simulink model "Requirements_Table"  (R2022a)
settings: Solver=FixedStepAuto  StartTime=0.0  StopTime=10.0  FixedStep=1e-3  RelTol=1e-3  EnableMultiTasking=on
settings Model: ExtModeTrigDuration=5  Creator=sabri  LastModifiedBy=Tim
settings SolverCC: AlgebraicLoopSolver=TrustRegion
settings OptimizationCC: EnhancedBackFolding=on  PassReuseOutputArgsAs=Individual arguments  ZeroExternalMemoryAtStartup=off  ZeroInternalMemoryAtStartup=off  MaxStackSize=64  OptimizeBlockOrder=speed  DifferentSizesBufferReuse=on  OptimizationCustomize=off  EfficientTunableParamExpr=on
settings DebuggingCC: ParameterTunabilityLossMsg=error  UnconnectedInputMsg=warning  UnconnectedOutputMsg=warning  UnconnectedLineMsg=warning  SFMachineParentedDataDiag=warning
settings HardwareCC: ProdBitPerPointer=32  ProdBitPerSizeT=32  ProdBitPerPtrDiffT=32  ProdLargestAtomicInteger=Long  ProdLargestAtomicFloat=Double  ProdWordSize=32  ProdHWDeviceType=ARM Compatible->ARM Cortex
settings SFSimCC: MATLABDynamicMemAlloc=off
settings RTWCC: SystemTargetFile=ert.tlc  HardwareBoard=NXP FRDM-K64F  TLCOptions="-aInlineSetEventsForThisBaseRateFcn=TLC_FALSE -aSuppressMultiTaskScheduler=TLC_FALSE  -aRateBasedStepFcn=0"  TemplateMakefile=ert_default_tmf  Toolchain=GNU Tools for ARM Embedded Processors
settings CodeAppCC: ForceParamTrailComments=on  IgnoreCustomStorageClasses=off  OperatorAnnotations=on  SimulinkDataObjDesc=on  SFDataObjDesc=on  InsertBlockDesc=on

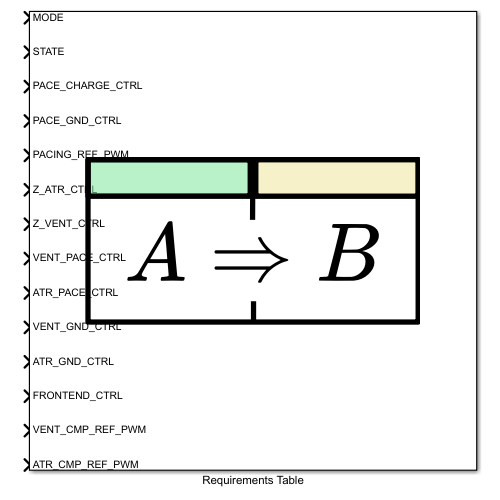
[thumbnail: Simulink's stored preview of the top-level diagram]
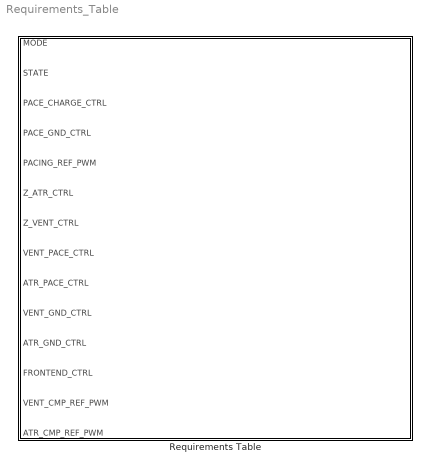
== system Requirements_Table ==
  Requirements Table : Requirements Table  TreatAsAtomicUnit=on

== stateflow chart Requirements_Table/Requirements Table ==
  (default) -> (junction 1073754062)
  (junction 1073754062) -> (junction 1073754063) : {
      | % SF_REQ_REV_07
      | }
  (junction 1073754063) -> (junction 1073754065) : {
      | % HEADER_ASSIGNMENTS
      |
      | }
  (junction 1073754065) -> (junction 1073754067) : {
      | % START_A_4
      | }
  (junction 1073754067) -> (junction 1073754069) : {
      | }
  (junction 1073754069) -> (junction 1073754071)
  (junction 1073754071) -> (junction 1073754073) : {
      | }
  (junction 1073754073) -> (junction 1073754075) : {
      | % END_A_4
      | }
  (junction 1073754075) -> (junction 1073754077) : {
      | % START_R_1
      | }
  (junction 1073754077) -> (junction 1073754079) : {
      | }
  (junction 1073754079) -> (junction 1073754081)
  (junction 1073754081) -> (junction 1073754083) [order 1] : [(((MODE) == (1)))]
  (junction 1073754081) -> (junction 1073754125) [order 2]
  (junction 1073754083) -> (junction 1073754085) : {
      | reqtable_postcondition((((FRONTEND_CTRL) == (0))), 'R:1');
      |
      |
      | }
  (junction 1073754085) -> (junction 1073754087) : {
      | }
  (junction 1073754087) -> (junction 1073754089) : {
      | % START_R_10
      | }
  (junction 1073754089) -> (junction 1073754091) : {
      | }
  (junction 1073754091) -> (junction 1073754093)
  (junction 1073754093) -> (junction 1073754095) [order 1] : [(((STATE) == (1)))]
  (junction 1073754093) -> (junction 1073754101) [order 2]
  (junction 1073754095) -> (junction 1073754097) : {
      | reqtable_postcondition((((PACE_CHARGE_CTRL) == (0))) && (((PACE_GND_CTRL) == (1))) && (((PACING_REF_PWM) == (vent_amp))) && (((Z_ATR_CTRL) == (0))) && (((Z_VENT_CTRL) == (0))) && (((VENT_PACE_CTRL) == (1))) && (((ATR_PACE_CTRL) == (0))) && (((VENT_GND_CTRL) == (0))) && (((ATR_GND_CTRL) == (0))), 'R:1.1');
      |
      |
      | }
  (junction 1073754097) -> (junction 1073754099) : {
      | }
  (junction 1073754099) -> (junction 1073754101)
  (junction 1073754101) -> (junction 1073754103)
  (junction 1073754103) -> (junction 1073754105) : {
      | % END_R_10
      | }
  (junction 1073754105) -> (junction 1073754107) : {
      | % START_R_16
      | }
  (junction 1073754107) -> (junction 1073754109) : {
      | }
  (junction 1073754109) -> (junction 1073754111)
  (junction 1073754111) -> (junction 1073754113) [order 1] : [(((STATE) == (0)))]
  (junction 1073754111) -> (junction 1073754119) [order 2]
  (junction 1073754113) -> (junction 1073754115) : {
      | reqtable_postcondition((((PACE_CHARGE_CTRL) == (1))) && (((PACE_GND_CTRL) == (1))) && (((PACING_REF_PWM) == (vent_amp))) && (((Z_ATR_CTRL) == (0))) && (((Z_VENT_CTRL) == (0))) && (((VENT_PACE_CTRL) == (0))) && (((ATR_PACE_CTRL) == (0))) && (((VENT_GND_CTRL) == (1))) && (((ATR_GND_CTRL) == (0))), 'R:1.2');
      |
      |
      | }
  (junction 1073754115) -> (junction 1073754117) : {
      | }
  (junction 1073754117) -> (junction 1073754119)
  (junction 1073754119) -> (junction 1073754121)
  (junction 1073754121) -> (junction 1073754123) : {
      | % END_R_16
      | }
  (junction 1073754123) -> (junction 1073754125)
  (junction 1073754125) -> (junction 1073754127)
  (junction 1073754127) -> (junction 1073754129) : {
      | % END_R_1
      | }
  (junction 1073754129) -> (junction 1073754131) : {
      | % START_R_7
      | }
  (junction 1073754131) -> (junction 1073754133) : {
      | }
  (junction 1073754133) -> (junction 1073754135)
  (junction 1073754135) -> (junction 1073754137) [order 1] : [(((MODE) == (2)))]
  (junction 1073754135) -> (junction 1073754179) [order 2]
  (junction 1073754137) -> (junction 1073754139) : {
      | reqtable_postcondition((((FRONTEND_CTRL) == (0))), 'R:2');
      |
      |
      | }
  (junction 1073754139) -> (junction 1073754141) : {
      | }
  (junction 1073754141) -> (junction 1073754143) : {
      | % START_R_19
      | }
  (junction 1073754143) -> (junction 1073754145) : {
      | }
  (junction 1073754145) -> (junction 1073754147)
  (junction 1073754147) -> (junction 1073754149) [order 1] : [(((STATE) == (1)))]
  (junction 1073754147) -> (junction 1073754155) [order 2]
  (junction 1073754149) -> (junction 1073754151) : {
      | reqtable_postcondition((((PACE_CHARGE_CTRL) == (0))) && (((PACE_GND_CTRL) == (1))) && (((PACING_REF_PWM) == (atr_amp))) && (((Z_ATR_CTRL) == (0))) && (((Z_VENT_CTRL) == (0))) && (((VENT_PACE_CTRL) == (0))) && (((ATR_PACE_CTRL) == (1))) && (((VENT_GND_CTRL) == (0))) && (((ATR_GND_CTRL) == (0))), 'R:2.1');
      |
      |
      | }
  (junction 1073754151) -> (junction 1073754153) : {
      | }
  (junction 1073754153) -> (junction 1073754155)
  (junction 1073754155) -> (junction 1073754157)
  (junction 1073754157) -> (junction 1073754159) : {
      | % END_R_19
      | }
  (junction 1073754159) -> (junction 1073754161) : {
      | % START_R_25
      | }
  (junction 1073754161) -> (junction 1073754163) : {
      | }
  (junction 1073754163) -> (junction 1073754165)
  (junction 1073754165) -> (junction 1073754167) [order 1] : [(((STATE) == (0)))]
  (junction 1073754165) -> (junction 1073754173) [order 2]
  (junction 1073754167) -> (junction 1073754169) : {
      | reqtable_postcondition((((PACE_CHARGE_CTRL) == (1))) && (((PACE_GND_CTRL) == (1))) && (((PACING_REF_PWM) == (atr_amp))) && (((Z_ATR_CTRL) == (0))) && (((Z_VENT_CTRL) == (0))) && (((VENT_PACE_CTRL) == (0))) && (((ATR_PACE_CTRL) == (0))) && (((VENT_GND_CTRL) == (0))) && (((ATR_GND_CTRL) == (1))), 'R:2.2');
      |
      |
      | }
  (junction 1073754169) -> (junction 1073754171) : {
      | }
  (junction 1073754171) -> (junction 1073754173)
  (junction 1073754173) -> (junction 1073754175)
  (junction 1073754175) -> (junction 1073754177) : {
      | % END_R_25
      | }
  (junction 1073754177) -> (junction 1073754179)
  (junction 1073754179) -> (junction 1073754181)
  (junction 1073754181) -> (junction 1073754183) : {
      | % END_R_7
      | }
  (junction 1073754183) -> (junction 1073754185) : {
      | % START_R_28
      | }
  (junction 1073754185) -> (junction 1073754187) : {
      | }
  (junction 1073754187) -> (junction 1073754189)
  (junction 1073754189) -> (junction 1073754191) [order 1] : [(((MODE) == (3)))]
  (junction 1073754189) -> (junction 1073754251) [order 2]
  (junction 1073754191) -> (junction 1073754193) : {
      |
      |
      | }
  (junction 1073754193) -> (junction 1073754195) : {
      | }
  (junction 1073754195) -> (junction 1073754197) : {
      | % START_R_34
      | }
  (junction 1073754197) -> (junction 1073754199) : {
      | }
  (junction 1073754199) -> (junction 1073754201)
  (junction 1073754201) -> (junction 1073754203) [order 1] : [(((STATE) == (1)))]
  (junction 1073754201) -> (junction 1073754209) [order 2]
  (junction 1073754203) -> (junction 1073754205) : {
      | reqtable_postcondition((((PACE_CHARGE_CTRL) == (0))) && (((PACE_GND_CTRL) == (1))) && (((PACING_REF_PWM) == (vent_amp))) && (((Z_ATR_CTRL) == (0))) && (((Z_VENT_CTRL) == (0))) && (((VENT_PACE_CTRL) == (1))) && (((ATR_PACE_CTRL) == (0))) && (((VENT_GND_CTRL) == (0))) && (((ATR_GND_CTRL) == (0))), 'R:3.1');
      |
      |
      | }
  (junction 1073754205) -> (junction 1073754207) : {
      | }
  (junction 1073754207) -> (junction 1073754209)
  (junction 1073754209) -> (junction 1073754211)
  (junction 1073754211) -> (junction 1073754213) : {
      | % END_R_34
      | }
  (junction 1073754213) -> (junction 1073754215) : {
      | % START_R_37
      | }
  (junction 1073754215) -> (junction 1073754217) : {
      | }
  (junction 1073754217) -> (junction 1073754219)
  (junction 1073754219) -> (junction 1073754221) [order 1] : [(((STATE) == (0)))]
  (junction 1073754219) -> (junction 1073754227) [order 2]
  (junction 1073754221) -> (junction 1073754223) : {
      | reqtable_postcondition((((PACE_CHARGE_CTRL) == (1))) && (((PACE_GND_CTRL) == (1))) && (((PACING_REF_PWM) == (vent_amp))) && (((Z_ATR_CTRL) == (0))) && (((Z_VENT_CTRL) == (0))) && (((VENT_PACE_CTRL) == (0))) && (((ATR_PACE_CTRL) == (0))) && (((VENT_GND_CTRL) == (1))) && (((ATR_GND_CTRL) == (0))) && (((FRONTEND_CTRL) == (1))), 'R:3.2');
      |
      |
      | }
  (junction 1073754223) -> (junction 1073754225) : {
      | }
  (junction 1073754225) -> (junction 1073754227)
  (junction 1073754227) -> (junction 1073754229)
  (junction 1073754229) -> (junction 1073754231) : {
      | % END_R_37
      | }
  (junction 1073754231) -> (junction 1073754233) : {
      | % START_R_40
      | }
  (junction 1073754233) -> (junction 1073754235) : {
      | }
  (junction 1073754235) -> (junction 1073754237)
  (junction 1073754237) -> (junction 1073754239) [order 1] : [(((STATE) == (2)))]
  (junction 1073754237) -> (junction 1073754245) [order 2]
  (junction 1073754239) -> (junction 1073754241) : {
      | reqtable_postcondition((((PACE_CHARGE_CTRL) == (1))) && (((PACE_GND_CTRL) == (1))) && (((PACING_REF_PWM) == (vent_amp))) && (((Z_ATR_CTRL) == (0))) && (((Z_VENT_CTRL) == (0))) && (((VENT_PACE_CTRL) == (0))) && (((ATR_PACE_CTRL) == (0))) && (((VENT_GND_CTRL) == (1))) && (((ATR_GND_CTRL) == (0))) && (((FRONTEND_CTRL) == (0))), 'R:3.3');
      |
      |
      | }
  (junction 1073754241) -> (junction 1073754243) : {
      | }
  (junction 1073754243) -> (junction 1073754245)
  (junction 1073754245) -> (junction 1073754247)
  (junction 1073754247) -> (junction 1073754249) : {
      | % END_R_40
      | }
  (junction 1073754249) -> (junction 1073754251)
  (junction 1073754251) -> (junction 1073754253)
  (junction 1073754253) -> (junction 1073754255) : {
      | % END_R_28
      | }
  (junction 1073754255) -> (junction 1073754257) : {
      | % START_R_31
      | }
  (junction 1073754257) -> (junction 1073754259) : {
      | }
  (junction 1073754259) -> (junction 1073754261)
  (junction 1073754261) -> (junction 1073754263) [order 1] : [(((MODE) == (4)))]
  (junction 1073754261) -> (junction 1073754323) [order 2]
  (junction 1073754263) -> (junction 1073754265) : {
      |
      |
      | }
  (junction 1073754265) -> (junction 1073754267) : {
      | }
  (junction 1073754267) -> (junction 1073754269) : {
      | % START_R_52
      | }
  (junction 1073754269) -> (junction 1073754271) : {
      | }
  (junction 1073754271) -> (junction 1073754273)
  (junction 1073754273) -> (junction 1073754275) [order 1] : [(((STATE) == (1)))]
  (junction 1073754273) -> (junction 1073754281) [order 2]
  (junction 1073754275) -> (junction 1073754277) : {
      | reqtable_postcondition((((PACE_CHARGE_CTRL) == (0))) && (((PACE_GND_CTRL) == (1))) && (((PACING_REF_PWM) == (atr_amp))) && (((Z_ATR_CTRL) == (0))) && (((Z_VENT_CTRL) == (0))) && (((VENT_PACE_CTRL) == (0))) && (((ATR_PACE_CTRL) == (1))) && (((VENT_GND_CTRL) == (0))) && (((ATR_GND_CTRL) == (0))), 'R:4.1');
      |
      |
      | }
  (junction 1073754277) -> (junction 1073754279) : {
      | }
  (junction 1073754279) -> (junction 1073754281)
  (junction 1073754281) -> (junction 1073754283)
  (junction 1073754283) -> (junction 1073754285) : {
      | % END_R_52
      | }
  (junction 1073754285) -> (junction 1073754287) : {
      | % START_R_55
      | }
  (junction 1073754287) -> (junction 1073754289) : {
      | }
  (junction 1073754289) -> (junction 1073754291)
  (junction 1073754291) -> (junction 1073754293) [order 1] : [(((STATE) == (0)))]
  (junction 1073754291) -> (junction 1073754299) [order 2]
  (junction 1073754293) -> (junction 1073754295) : {
      | reqtable_postcondition((((PACE_CHARGE_CTRL) == (1))) && (((PACE_GND_CTRL) == (1))) && (((PACING_REF_PWM) == (atr_amp))) && (((Z_ATR_CTRL) == (0))) && (((Z_VENT_CTRL) == (0))) && (((VENT_PACE_CTRL) == (0))) && (((ATR_PACE_CTRL) == (0))) && (((VENT_GND_CTRL) == (0))) && (((ATR_GND_CTRL) == (1))) && (((FRONTEND_CTRL) == (1))), 'R:4.2');
      |
      |
      | }
  (junction 1073754295) -> (junction 1073754297) : {
      | }
  (junction 1073754297) -> (junction 1073754299)
  (junction 1073754299) -> (junction 1073754301)
  (junction 1073754301) -> (junction 1073754303) : {
      | % END_R_55
      | }
  (junction 1073754303) -> (junction 1073754305) : {
      | % START_R_58
      | }
  (junction 1073754305) -> (junction 1073754307) : {
      | }
  (junction 1073754307) -> (junction 1073754309)
  (junction 1073754309) -> (junction 1073754311) [order 1] : [(((STATE) == (2)))]
  (junction 1073754309) -> (junction 1073754317) [order 2]
  (junction 1073754311) -> (junction 1073754313) : {
      | reqtable_postcondition((((PACE_CHARGE_CTRL) == (1))) && (((PACE_GND_CTRL) == (1))) && (((PACING_REF_PWM) == (atr_amp))) && (((Z_ATR_CTRL) == (0))) && (((Z_VENT_CTRL) == (0))) && (((VENT_PACE_CTRL) == (0))) && (((ATR_PACE_CTRL) == (0))) && (((VENT_GND_CTRL) == (0))) && (((ATR_GND_CTRL) == (1))) && (((FRONTEND_CTRL) == (0))), 'R:4.3');
      |
      |
      | }
  (junction 1073754313) -> (junction 1073754315) : {
      | }
  (junction 1073754315) -> (junction 1073754317)
  (junction 1073754317) -> (junction 1073754319)
  (junction 1073754319) -> (junction 1073754321) : {
      | % END_R_58
      | }
  (junction 1073754321) -> (junction 1073754323)
  (junction 1073754323) -> (junction 1073754325)
  (junction 1073754325) -> (junction 1073754327) : {
      | % END_R_31
      | }
  data: MODE input; STATE input; PACE_CHARGE_CTRL input; PACE_GND_CTRL input; PACING_REF_PWM input; Z_ATR_CTRL input; Z_VENT_CTRL input; VENT_PACE_CTRL input; ATR_PACE_CTRL input; VENT_GND_CTRL input; ATR_GND_CTRL input; FRONTEND_CTRL input; VENT_CMP_REF_PWM input; ATR_CMP_REF_PWM input
